simulink model "DSTR"  (R2023a)
settings: Solver=FixedStepAuto  StartTime=t_0  StopTime=t_f  FixedStep=dt  RelTol=1e-3
values from neighbouring files (symbols this model uses):
  A = H.Denominator{1}    [example7.m]
  A0 = 1    [example7.m]
  Am = Hm.Denominator{1}    [example7.m]
  B = H.Numerator{1}    [example7.m]
  Bm = sum(Am)    [example7.m]
  d0 = 2    [example7.m]
  h = 0.5    [example4.m]    (also in example7.m)
  l = 1    [example7.m]
  P0 = diag([100 100 1 1])    [example4.m]    (also in example7.m = 10*eye(4))
  theta0 = [0; 0; 0.01; 0.2]    [example4.m]    (also in example7.m = [1 0 0 0]')
libraries: simulink x2
settings Model: Creator=Mmoha  LastModifiedBy=Mmoha

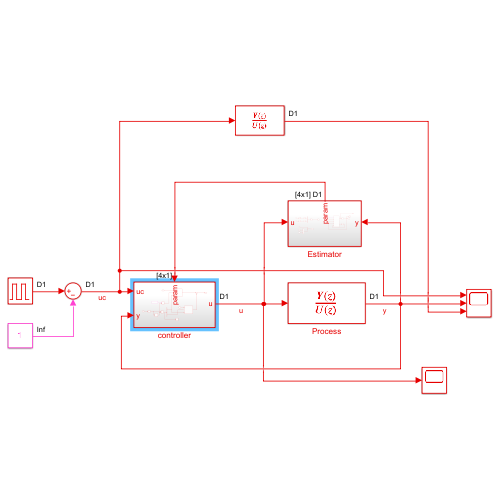
[thumbnail: Simulink's stored preview of the top-level diagram]
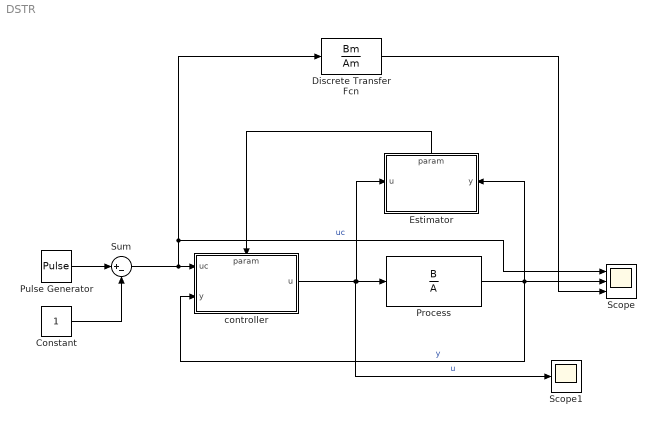
== system DSTR ==
  Constant : Constant
  Discrete Transfer Fcn : DiscreteTransferFcn  Numerator=Bm  Denominator=Am  SampleTime=h  a0EqualsOne=on
  Estimator : Subsystem
      settings: PortSchema="{\"entries\":[{\"content\":{\"sides\":[{\"content\":{\"connectorIds\":[\"In1\"]},\"type\":\"ConnectorPlacement.EquallySpacedRectSide\",\"uuid\":\"d59c4060-ca18-4c06-9040-48d101e58fef\"},{\"content\":{\"connectorIds\":[\"In2\"],\"side\":\"RIGHT\"},\"type\":\"ConnectorPlacement.EquallySpacedRectSide\",\"uuid\":\"6d166754-2246-4e16-bafc-8a94baa0622a\"},{\"content\":{\"connectorIds\":[\"Out1\"],\"side\":\"TOP\"},\"type\":\"ConnectorPlacement.EquallySpacedRectSide\",\"uuid\":\"f832d6d8-6c2a-4217-853e-56f1c457f30a\"}]},\"type\":\"ConnectorPlacement.EquallySpacedConnector\",\"uuid\":\"75872c2c-de78-4943-95d8-62516a499510\"}],\"packageUris\":[\"http://schema.mathworks.com/mf0/Connector/R2020b\"],\"version\":\"1.0\"}"
  Process : DiscreteTransferFcn  Numerator=B  Denominator=A  SampleTime=h  a0EqualsOne=on
  Pulse Generator : DiscretePulseGenerator  PulseType=Time based  Amplitude=2  Period=50  PulseWidth=50
  Scope : Scope  NumInputPorts=3
  Scope1 : Scope
  Sum : Sum  Inputs=|+-
  controller : Subsystem
      settings: PortSchema="{\"entries\":[{\"content\":{\"sides\":[{\"content\":{\"connectorIds\":[\"In1\",\"In2\"]},\"type\":\"ConnectorPlacement.EquallySpacedRectSide\",\"uuid\":\"d59c4060-ca18-4c06-9040-48d101e58fef\"},{\"content\":{\"connectorIds\":[\"Out1\"],\"side\":\"RIGHT\"},\"type\":\"ConnectorPlacement.EquallySpacedRectSide\",\"uuid\":\"6d166754-2246-4e16-bafc-8a94baa0622a\"},{\"content\":{\"connectorIds\":[\"In3\"],\"side\":\"TOP\"},\"type\":\"ConnectorPlacement.EquallySpacedRectSide\",\"uuid\":\"f832d6d8-6c2a-4217-853e-56f1c457f30a\"}]},\"type\":\"ConnectorPlacement.EquallySpacedConnector\",\"uuid\":\"75872c2c-de78-4943-95d8-62516a499510\"}],\"packageUris\":[\"http://schema.mathworks.com/mf0/Connector/R2020b\"],\"version\":\"1.0\"}"
  wires:
  Pulse Generator/1 -> Sum/1
  Constant/1 -> Sum/2
  Sum/1 -> Discrete Transfer Fcn/1, Scope/1, controller/1(uc)  "uc"
  controller/1(u) -> Scope1/1, Estimator/1(u), Process/1  "u"
  Process/1 -> Estimator/2(y), Scope/2, controller/2(y)  "y"
  Estimator/1(param) -> controller/3(param)
  Discrete Transfer Fcn/1 -> Scope/3

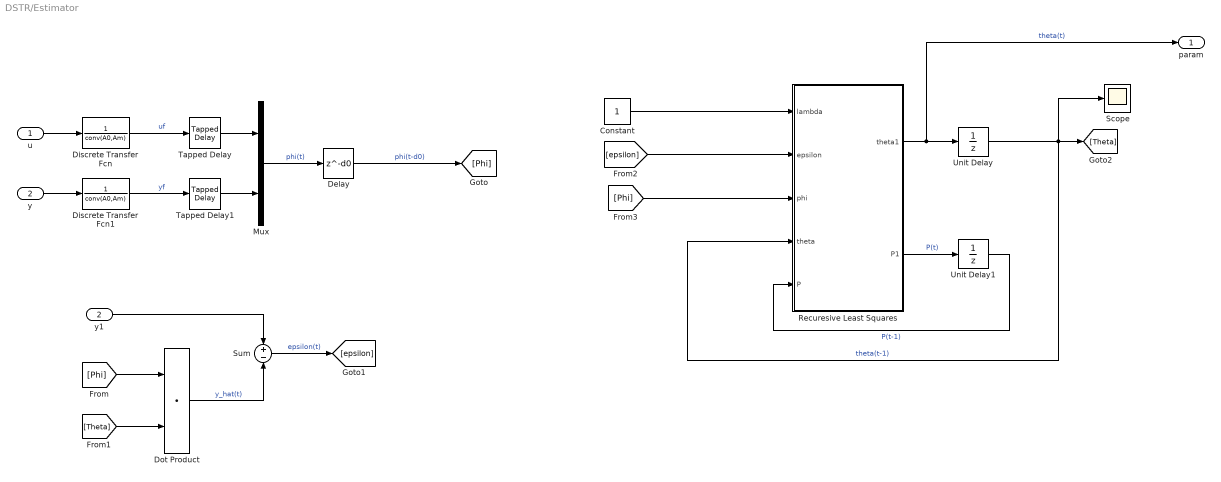
== system DSTR/Estimator ==
  u : Inport
  y : Inport  Port=2
  Constant : Constant
  Delay : Delay  DelayLength=d0  SampleTime=h
  Discrete Transfer Fcn : DiscreteTransferFcn  Denominator=conv(A0,Am)  SampleTime=h
  Discrete Transfer Fcn1 : DiscreteTransferFcn  Denominator=conv(A0,Am)  SampleTime=h
  Dot Product : DotProduct  OutDataTypeStr=Inherit: Inherit via internal rule
  Mux : Mux  Inputs=2
  Recuresive Least Squares : MATLAB Function  TreatAsAtomicUnit=on
  Scope : Scope
  Sum : Sum  Inputs=+|-
  Tapped Delay : simulink/Discrete/Tapped Delay  vinit=0.0  samptime=h  NumDelays=l  DelayOrder=Newest  includeCurrent=on
  Tapped Delay1 : simulink/Discrete/Tapped Delay  vinit=0.0  samptime=h  NumDelays=l  DelayOrder=Newest  includeCurrent=on
  Unit Delay : UnitDelay  InitialCondition=theta0  SampleTime=h  HasFrameUpgradeWarning=on
  Unit Delay1 : UnitDelay  InitialCondition=P0  SampleTime=h  HasFrameUpgradeWarning=on
  y1 : InportShadow  Port=2
  param : Outport
  wires:
  u/1 -> Discrete Transfer Fcn/1
  y/1 -> Discrete Transfer Fcn1/1
  Discrete Transfer Fcn/1 -> Tapped Delay/1  "uf"
  Discrete Transfer Fcn1/1 -> Tapped Delay1/1  "yf"
  Tapped Delay/1 -> Mux/1
  Tapped Delay1/1 -> Mux/2
  Mux/1 -> Delay/1  "phi(t)"
  Delay/1 -> [Phi]  "phi(t-d0)"
  [Phi] -> Dot Product/1
  [Theta] -> Dot Product/2
  Dot Product/1 -> Sum/2  "y_hat(t)"
  y1/1 -> Sum/1
  Sum/1 -> [epsilon]  "epsilon(t)"
  Recuresive Least Squares/1(theta1) -> param/1, Unit Delay/1  "theta(t)"
  Recuresive Least Squares/2(P1) -> Unit Delay1/1  "P(t)"
  Unit Delay/1 -> Recuresive Least Squares/4(theta), Scope/1, [Theta]  "theta(t-1)"
  Unit Delay1/1 -> Recuresive Least Squares/5(P)  "P(t-1)"
  [epsilon] -> Recuresive Least Squares/2(epsilon)
  Constant/1 -> Recuresive Least Squares/1(lambda)
  [Phi] -> Recuresive Least Squares/3(phi)

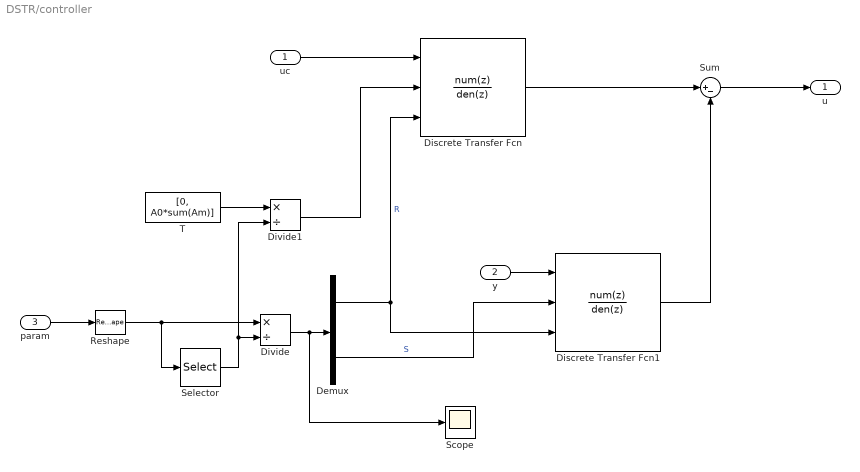
== system DSTR/controller ==
  uc : Inport
  y : Inport  Port=2
  param : Inport  Port=3
  Demux : Demux  Outputs=2
  Discrete Transfer Fcn : DiscreteTransferFcn  NumeratorSource=Input port  DenominatorSource=Input port  SampleTime=h  a0EqualsOne=on
      settings: InputPortMap=u0,p1,p3
  Discrete Transfer Fcn1 : DiscreteTransferFcn  NumeratorSource=Input port  DenominatorSource=Input port  SampleTime=h  a0EqualsOne=on
      settings: InputPortMap=u0,p1,p3
  Divide : Product  Inputs=*/
  Divide1 : Product  Inputs=*/
  Reshape : Reshape
  Scope : Scope
  Selector : Selector  InputPortWidth=4  IndexOptions=Index vector (dialog)  Indices=[1]  OutputSizes=1
  Sum : Sum  Inputs=|+-
  T : Constant  Value=[0, A0*sum(Am)]
  u : Outport
  wires:
  uc/1 -> Discrete Transfer Fcn/1
  param/1 -> Reshape/1
  Demux/1 -> Discrete Transfer Fcn/3, Discrete Transfer Fcn1/3  "R"
  Demux/2 -> Discrete Transfer Fcn1/2  "S"
  Selector/1 -> Divide/2, Divide1/2
  Divide/1 -> Scope/1, Demux/1
  T/1 -> Divide1/1
  Divide1/1 -> Discrete Transfer Fcn/2
  y/1 -> Discrete Transfer Fcn1/1
  Discrete Transfer Fcn/1 -> Sum/1
  Discrete Transfer Fcn1/1 -> Sum/2
  Sum/1 -> u/1
  Reshape/1 -> Divide/1, Selector/1

== matlab function DSTR/Estimator/Recuresive Least Squares ==
  data: lambda input size=1; theta1 output size=[4 1]; epsilon input size=1; phi input size=[4 1]; theta input size=[4 1]; P input size=[4 4]; P1 output size=[4 4]
function [theta1, P1] = rls(lambda, epsilon, phi, theta, P)
K = P * phi / (lambda + phi'*P*phi);
P1 = (eye(4) - K*phi') * P / lambda;
theta1 = theta + P1 * phi * epsilon;
